simulink model "MultiLoop_mode1"  (R2021b)
settings: Solver=ode45  StartTime=0.0  StopTime=72  FixedStep=Ts_base  MinStep=1e-6  RelTol=1e-6
PreLoadFcn:
  | Mode_1_Init
InitFcn:
  | hApp = TEP_app;
  | %hApp = fault_selection_App;
StartFcn:
  | disp('simulator')
  | blk = 'MultiLoop_mode1/TE Plant/Pressure';
  | event = 'PostOutputs';
  | listener = @(app, event) updateGUI(hApp);
  | h = add_exec_event_listener(blk, event, listener);
StopFcn:
  | %TEplot
undefined symbols (not defined in the file or in its folder): Eadj_0, r1_0, r4_0, r5_0, r6_0, r7_0, SP17_0, Ts_base, Ts_save, xmv10_0, xmv11_0
libraries: TElib x8
settings Model: Creator=ricker  LastModifiedBy=kaung
settings SolverCC: AlgebraicLoopSolver=TrustRegion
settings DataIOCC: LoadInitialState=on  SaveFinalState=on  SaveFormat=Structure  SignalLoggingSaveFormat=ModelDataLogs  SaveOutput=off  SignalLogging=off  SaveTime=off  ReturnWorkspaceOutputs=off  SignalLoggingName=sigsOut
settings OptimizationCC: InitFltsAndDblsToZero=on  LifeSpan=inf
settings DebuggingCC: SaveWithParameterizedLinksMsg=none  UnderspecifiedInitializationDetection=Classic  MergeDetectMultiDrivingBlocksExec=none  SignalResolutionControl=TryResolveAllWithWarning  MultiTaskDSMMsg=warning  MultiTaskCondExecSysMsg=none  FcnCallInpInsideContextMsg=warning  SFUnexpectedBacktrackingDiag=warning  SFNoUnconditionalDefaultTransitionDiag=warning  SFExecutionAtInitializationDiag=none  SFMachineParentedDataDiag=warning  ArithmeticOperatorsInVariantConditions=warning
settings HardwareCC: ProdBitPerPointer=32  ProdBitPerSizeT=32  ProdBitPerPtrDiffT=32  ProdLargestAtomicFloat=None  ProdIntDivRoundTo=Undefined  ProdEndianess=Unspecified  ProdWordSize=32  ProdHWDeviceType=32-bit Generic  TargetUnknown=on
settings ModelReferenceCC: PropagateSignalLabelsOutOfModel=off
settings SFSimCC: SimUseLocalCustomCode=off  CustomCodeUndefinedFunction=UseInterfaceOnly
settings RTWCC: RTWUseLocalCustomCode=off
settings CodeAppCC: StateflowObjectComments=on
settings GRTTargetCC: TargetFcnLib=ansi_tfl_tmw.mat  TargetLangStandard=C89/C90 (ANSI)  CombineOutputUpdateFcns=off  GRTInterface=on
settings ConfigComp: CovMetricSettings=dw  CovSaveCumulativeToWorkspaceVar=on  CovSaveSingleToWorkspaceVar=on  CovExternalEMLEnable=off  CovSFcnEnable=off

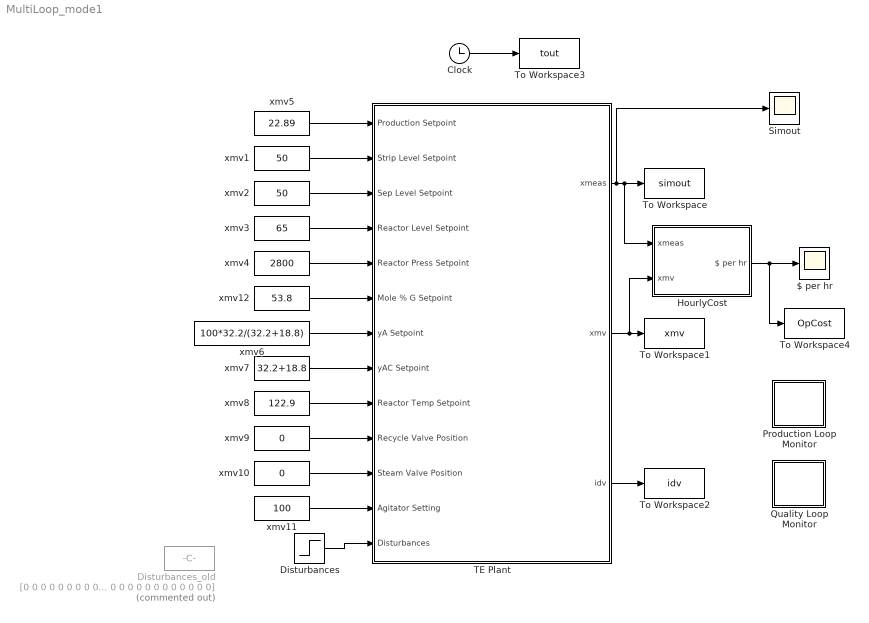
== system MultiLoop_mode1 ==
  $ per hr : Scope
  Clock : Clock
  Disturbances : Step  Time=0  Before=[0 0 0 0 0 0 0 0 0 0 0 0 0 0 0 0 0 0 0 0 0 0 0 0 0 0 0 0]  After=[1 0 0 0 0 0 0 0 0 0 0 0 0 0 0 0 0 0 0 0 0 0 0 0 0 0 0 0]  SampleTime=0
  Disturbances_old : Constant  Commented=on  Value=[0 0 0 0 0 0 0 0 0 0 0 0 0 0 0 0 0 0 0 0 0 0 0 0 0 0 0 0]
  HourlyCost : Subsystem
  Production Loop Monitor : Subsystem
  Quality Loop Monitor : Subsystem
  Simout : Scope
  TE Plant : Subsystem
  To Workspace : ToWorkspace  VariableName=simout  SampleTime=Ts_save
  To Workspace1 : ToWorkspace  VariableName=xmv  SampleTime=Ts_save
  To Workspace2 : ToWorkspace  VariableName=idv  SampleTime=Ts_save
  To Workspace3 : ToWorkspace  VariableName=tout  SampleTime=Ts_save
  To Workspace4 : ToWorkspace  VariableName=OpCost  SampleTime=Ts_save
  xmv1 : Constant  Value=50
  xmv10 : Constant  Value=0
  xmv11 : Constant  Value=100
  xmv12 : Constant  Value=53.8
  xmv2 : Constant  Value=50
  xmv3 : Constant  Value=65
  xmv4 : Constant  Value=2800
  xmv5 : Constant  Value=22.89
  xmv6 : Constant  Value=100*32.2/(32.2+18.8)
  xmv7 : Constant  Value=32.2+18.8
  xmv8 : Constant  Value=122.9
  xmv9 : Constant  Value=0
  wires:
  TE Plant/1(xmeas) -> Simout/1, To Workspace/1, HourlyCost/1(xmeas)
  xmv1/1 -> TE Plant/2(Strip Level Setpoint)
  xmv2/1 -> TE Plant/3(Sep Level Setpoint)
  xmv3/1 -> TE Plant/4(Reactor Level Setpoint)
  xmv4/1 -> TE Plant/5(Reactor Press Setpoint)
  xmv8/1 -> TE Plant/9(Reactor Temp Setpoint)
  xmv6/1 -> TE Plant/7(yA Setpoint)
  xmv7/1 -> TE Plant/8(yAC Setpoint)
  TE Plant/2(xmv) -> To Workspace1/1, HourlyCost/2(xmv)
  TE Plant/3(idv) -> To Workspace2/1
  Clock/1 -> To Workspace3/1
  HourlyCost/1($ per hr) -> $ per hr/1, To Workspace4/1
  xmv9/1 -> TE Plant/10(Recycle Valve Position)
  xmv10/1 -> TE Plant/11(Steam Valve Position)
  xmv11/1 -> TE Plant/12(Agitator Setting)
  xmv12/1 -> TE Plant/6(Mole % G Setpoint)
  Disturbances/1 -> TE Plant/13(Disturbances)
  xmv5/1 -> TE Plant/1(Production Setpoint)

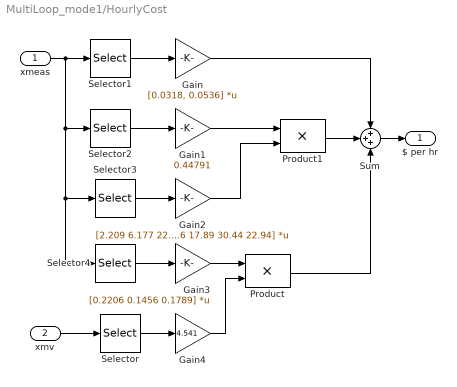
== system MultiLoop_mode1/HourlyCost ==
  xmeas : Inport  PortDimensions=41
  xmv : Inport  Port=2  PortDimensions=12
  Gain : Gain  Gain=[0.0318, 0.0536]  Multiplication=Matrix(K*u)  SaturateOnIntegerOverflow=on  OutDataTypeStr=Inherit: Same as input  ParamDataTypeStr=Inherit: Same as input
  Gain1 : Gain  Gain=0.44791  SaturateOnIntegerOverflow=on  OutDataTypeStr=Inherit: Same as input  ParamDataTypeStr=Inherit: Same as input
  Gain2 : Gain  Gain=[2.209 6.177 22.06 14.56 17.89 30.44 22.94]  Multiplication=Matrix(K*u)  SaturateOnIntegerOverflow=on  OutDataTypeStr=Inherit: Same as input  ParamDataTypeStr=Inherit: Same as input
  Gain3 : Gain  Gain=[0.2206 0.1456 0.1789]  Multiplication=Matrix(K*u)  SaturateOnIntegerOverflow=on  OutDataTypeStr=Inherit: Same as input  ParamDataTypeStr=Inherit: Same as input
  Gain4 : Gain  Gain=4.541  SaturateOnIntegerOverflow=on  OutDataTypeStr=Inherit: Same as input  ParamDataTypeStr=Inherit: Same as input
  Product : Product  SaturateOnIntegerOverflow=on  OutDataTypeStr=Inherit: Same as first input
  Product1 : Product  SaturateOnIntegerOverflow=on  OutDataTypeStr=Inherit: Same as first input
  Selector : Selector  InputPortWidth=12  IndexOptions=Index vector (dialog)  Indices=8  OutputSizes=1
  Selector1 : Selector  InputPortWidth=41  IndexOptions=Index vector (dialog)  Indices=[19 20]  OutputSizes=1
  Selector2 : Selector  InputPortWidth=41  IndexOptions=Index vector (dialog)  Indices=[10]  OutputSizes=1
  Selector3 : Selector  InputPortWidth=41  IndexOptions=Index vector (dialog)  Indices=[29, 31:36]  OutputSizes=1
  Selector4 : Selector  InputPortWidth=41  IndexOptions=Index vector (dialog)  Indices=[37:39]  OutputSizes=1
  Sum : Sum  Inputs=+++  SaturateOnIntegerOverflow=on
  $ per hr : Outport
  wires:
  xmv/1 -> Selector/1
  xmeas/1 -> Selector1/1, Selector2/1, Selector3/1, Selector4/1
  Selector1/1 -> Gain/1
  Selector2/1 -> Gain1/1
  Selector3/1 -> Gain2/1
  Selector4/1 -> Gain3/1
  Selector/1 -> Gain4/1
  Gain3/1 -> Product/1
  Gain4/1 -> Product/2
  Sum/1 -> $ per hr/1
  Product/1 -> Sum/3
  Gain/1 -> Sum/1
  Product1/1 -> Sum/2
  Gain1/1 -> Product1/1
  Gain2/1 -> Product1/2

== system MultiLoop_mode1/Production Loop Monitor ==
  Mux2 : Mux  Inputs=2
  Production : Scope
  wires:
  Mux2/1 -> Production/1
  [xmeas17] -> Mux2/2
  [Prodsp] -> Mux2/1

== system MultiLoop_mode1/Quality Loop Monitor ==
  Mux2 : Mux  Inputs=2
  Quality : Scope
  wires:
  [PctGsp] -> Mux2/1
  [xmeas40] -> Mux2/2
  Mux2/1 -> Quality/1

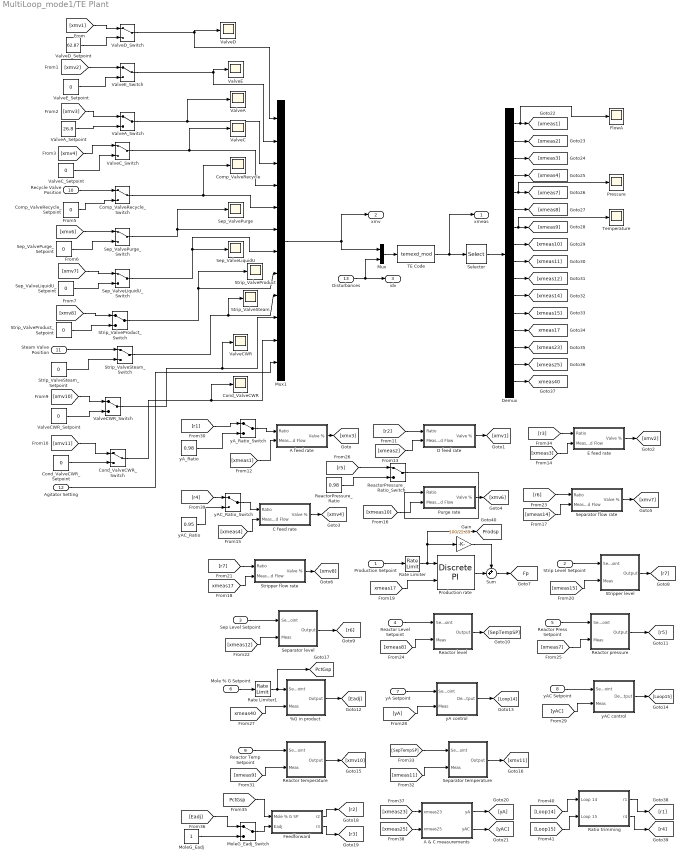
== system MultiLoop_mode1/TE Plant ==
  Production Setpoint : Inport
  Strip Level Setpoint : Inport  Port=2
  Sep Level Setpoint : Inport  Port=3
  Reactor Level Setpoint : Inport  Port=4
  Reactor Press Setpoint : Inport  Port=5
  Mole % G Setpoint : Inport  Port=6
  yA Setpoint : Inport  Port=7
  yAC Setpoint : Inport  Port=8
  Reactor Temp Setpoint : Inport  Port=9
  Recycle Valve Position : Inport  Port=10
  Steam Valve Position : Inport  Port=11
  Agitator Setting : Inport  Port=12
  Disturbances : Inport  Port=13
  %G in product : Subsystem  AncestorBlock=TElib/Discrete PI  mask{Kc=-0.4, Ti=100/60, Ts=Ts_base, x0=Eadj_0, Hi=inf, Lo=-inf}
  A & C measurements : Subsystem
  A feed rate : Subsystem
  C feed rate : Subsystem
  Comp_ValveRecycle : Scope
  Comp_ValveRecycle_Setpoint : Constant  Value=0
  Comp_ValveRecycle_Switch : ManualSwitch
  Cond_ValveCWR : Scope
  Cond_ValveCWR_Setpoint : Constant  Value=0
  Cond_ValveCWR_Switch : ManualSwitch
  D feed rate : Subsystem
  Demux : Demux  Outputs=16
      settings: DisplayOption=none
  E feed rate : Subsystem
  Feedforward : Subsystem
  FlowA : Scope
  Gain : Gain  Gain=100/22.89  SaturateOnIntegerOverflow=on  OutDataTypeStr=Inherit: Same as input  ParamDataTypeStr=Inherit: Same as input
  MoleG_Eadj : Constant
  MoleG_Eadj_Switch : ManualSwitch
  Mux : Mux  Inputs=2
  Mux1 : Mux  Inputs=12
  Pressure : Scope
  Production rate : TElib/Discrete PI  Kc=3.2  Ti=120/60  Ts=Ts_base  x0=0  Hi=30  Lo=-30
  Purge rate : Subsystem
  Rate Limiter : RateLimiter  RisingSlewLimit=0.3*22.95/24  FallingSlewLimit=-0.3*22.95/24
  Rate Limiter1 : RateLimiter  RisingSlewLimit=50/24  FallingSlewLimit=-50/24
  Ratio trimming : Subsystem
  Reactor level : Subsystem  AncestorBlock=TElib/Discrete PI  mask{Kc=0.8, Ti=60/60, Ts=Ts_base, x0=SP17_0, Hi=120, Lo=0}
  Reactor pressure : Subsystem  AncestorBlock=TElib/Discrete PI  mask{Kc=-1e-4, Ti=20/60, Ts=Ts_base, x0=r5_0, Hi=100, Lo=0}
  Reactor temperature : Subsystem  AncestorBlock=TElib/Discrete PI  mask{Kc=-8, Ti=7.5/60, Ts=Ts_base, x0=xmv10_0, Hi=100, Lo=0}
  ReactorPressure_Ratio : Constant  Value=0.98
  ReactorPressure_Ratio_Switch : ManualSwitch
  Selector : Selector  InputPortWidth=41  IndexOptions=Index vector (dialog)  Indices=[1:4, 7:12, 14, 15, 17, 23, 25, 40]  OutputSizes=1
  Sep_ValveLiquidU : Scope
  Sep_ValveLiquidU_Setpoint : Constant  Value=0
  Sep_ValveLiquidU_Switch : ManualSwitch
  Sep_ValvePurge : Scope
  Sep_ValvePurge_Setpoint : Constant  Value=0
  Sep_ValvePurge_Switch : ManualSwitch
  Separator flow rate : Subsystem
  Separator level : Subsystem  AncestorBlock=TElib/Discrete PI  mask{Kc=-1e-3, Ti=200/60, Ts=Ts_base, x0=r6_0, Hi=100, Lo=0}
  Separator temperature : Subsystem  AncestorBlock=TElib/Discrete PI  mask{Kc=-4, Ti=15/60, Ts=Ts_base, x0=xmv11_0, Hi=100, Lo=0}
  Strip_ValveProduct : Scope
  Strip_ValveProduct_Setpoint : Constant  Value=0
  Strip_ValveProduct_Switch : ManualSwitch
  Strip_ValveSteam : Scope
  Strip_ValveSteam_Setpoint : Constant  Value=0
  Strip_ValveSteam_Switch : ManualSwitch
  Stripper flow rate : Subsystem
  Stripper level : Subsystem  AncestorBlock=TElib/Discrete PI  mask{Kc=-2e-4, Ti=200/60, Ts=Ts_base, x0=r7_0, Hi=100, Lo=0}
  Sum : Sum  Inputs=++|  SaturateOnIntegerOverflow=on
  TE Code : S-Function  FunctionName=temexd_mod  SFunctionDeploymentMode=off  EnableBusSupport=off
  Temperature : Scope
  ValveA : Scope
  ValveA_Setpoint : Constant  Value=26.8
  ValveA_Switch : ManualSwitch
  ValveC : Scope
  ValveCWR : Scope
  ValveCWR_Setpoint : Constant  Value=0
  ValveCWR_Switch : ManualSwitch
  ValveC_Setpoint : Constant  Value=0
  ValveC_Switch : ManualSwitch
  ValveD : Scope
  ValveD_Setpoint : Constant  Value=62.87
  ValveD_Switch : ManualSwitch
  ValveE : Scope
  ValveE_Setpoint : Constant  Value=0
  ValveE_Switch : ManualSwitch
  yA control : Subsystem  AncestorBlock=TElib/Discrete PI/Vel PI  mask{Kc=2e-4, Ti=1, Ts=0.1}
  yAC control : Subsystem  AncestorBlock=TElib/Discrete PI/Vel PI  mask{Kc=3e-4, Ti=2, Ts=0.1}
  yAC_Ratio : Constant  Value=0.95
  yAC_Ratio_Switch : ManualSwitch
  yA_Ratio : Constant  Value=0.98
  yA_Ratio_Switch : ManualSwitch
  xmeas : Outport
  xmv : Outport  Port=2
  idv : Outport  Port=3
  tag scope: Fp=global, PctGsp=global, Prodsp=global, xmeas17=global, xmeas40=global
  wires:
  Mux/1 -> TE Code/1
  Disturbances/1 -> Mux/2, idv/1
  TE Code/1 -> xmeas/1, Selector/1
  [xmv1] -> ValveD_Switch/1
  Recycle Valve Position/1 -> Comp_ValveRecycle_Switch/1
  [xmv6] -> Sep_ValvePurge_Switch/1
  [xmv7] -> Sep_ValveLiquidU_Switch/1
  [xmv8] -> Strip_ValveProduct_Switch/1
  Steam Valve Position/1 -> Strip_ValveSteam_Switch/1
  [xmv10] -> ValveCWR_Switch/1
  [xmv11] -> Cond_ValveCWR_Switch/1
  Agitator Setting/1 -> Mux1/12
  A feed rate/1(Valve %) -> [xmv3]
  [xmeas1] -> A feed rate/2(Measured Flow)
  D feed rate/1(Valve %) -> [xmv1]
  [xmeas2] -> D feed rate/2(Measured Flow)
  E feed rate/1(Valve %) -> [xmv2]
  [xmeas3] -> E feed rate/2(Measured Flow)
  C feed rate/1(Valve %) -> [xmv4]
  [xmeas4] -> C feed rate/2(Measured Flow)
  Purge rate/1(Valve %) -> [xmv6]
  [xmeas10] -> Purge rate/2(Measured Flow)
  Separator flow rate/1(Valve %) -> [xmv7]
  [xmeas14] -> Separator flow rate/2(Measured Flow)
  Stripper flow rate/1(Valve %) -> [xmv8]
  [xmeas17] -> Stripper flow rate/2(Measured Flow)
  [xmeas17] -> Production rate/2
  [xmeas15] -> Stripper level/2(Meas)
  Strip Level Setpoint/1 -> Stripper level/1(Setpoint)
  Stripper level/1(Output) -> [r7]
  [r7] -> Stripper flow rate/1(Ratio)
  [xmeas12] -> Separator level/2(Meas)
  Sep Level Setpoint/1 -> Separator level/1(Setpoint)
  Separator level/1(Output) -> [r6]
  [r6] -> Separator flow rate/1(Ratio)
  [xmeas8] -> Reactor level/2(Meas)
  Reactor Level Setpoint/1 -> Reactor level/1(Setpoint)
  Reactor level/1(Output) -> [SepTempSP]
  [xmeas7] -> Reactor pressure/2(Meas)
  Reactor Press Setpoint/1 -> Reactor pressure/1(Setpoint)
  Reactor pressure/1(Output) -> [r5]
  [r5] -> ReactorPressure_Ratio_Switch/1
  [xmeas40] -> %G in product/2(Meas)
  %G in product/1(Output) -> [Eadj]
  [yA] -> yA control/2(Meas)
  yA Setpoint/1 -> yA control/1(Setpoint)
  yA control/1(Delta Output) -> [Loop14]
  [yAC] -> yAC control/2(Meas)
  yAC Setpoint/1 -> yAC control/1(Setpoint)
  yAC control/1(Delta Output) -> [Loop15]
  [r1] -> yA_Ratio_Switch/1
  [xmeas9] -> Reactor temperature/2(Meas)
  Reactor Temp Setpoint/1 -> Reactor temperature/1(Setpoint)
  Reactor temperature/1(Output) -> [xmv10]
  [xmeas11] -> Separator temperature/2(Meas)
  [SepTempSP] -> Separator temperature/1(Setpoint)
  Separator temperature/1(Output) -> [xmv11]
  [r3] -> E feed rate/1(Ratio)
  [PctGsp] -> Feedforward/1(Mole % G SP)
  [Eadj] -> MoleG_Eadj_Switch/1
  Feedforward/1(r2) -> [r2]
  Feedforward/2(r3) -> [r3]
  [xmeas23] -> A & C measurements/1(xmeas23)
  [xmeas25] -> A & C measurements/2(xmeas25)
  A & C measurements/1(yA) -> [yA]
  A & C measurements/2(yAC) -> [yAC]
  Mux1/1 -> Mux/1, xmv/1
  Selector/1 -> Demux/1
  Demux/1 -> FlowA/1, [xmeas1]
  Demux/2 -> [xmeas2]
  Demux/3 -> [xmeas3]
  Demux/4 -> [xmeas4]
  Demux/5 -> [xmeas7], Pressure/1
  Demux/6 -> [xmeas8]
  Demux/7 -> [xmeas9], Temperature/1
  Demux/8 -> [xmeas10]
  Demux/9 -> [xmeas11]
  Demux/10 -> [xmeas12]
  Demux/11 -> [xmeas14]
  Demux/12 -> [xmeas15]
  Demux/13 -> [xmeas17]
  Demux/14 -> [xmeas23]
  Demux/15 -> [xmeas25]
  Demux/16 -> [xmeas40]
  [r4] -> yAC_Ratio_Switch/1
  [Loop14] -> Ratio trimming/1(Loop 14)
  [Loop15] -> Ratio trimming/2(Loop 15)
  Ratio trimming/1(r1) -> [r1]
  Ratio trimming/2(r4) -> [r4]
  Production Setpoint/1 -> Rate Limiter/1
  Rate Limiter/1 -> Production rate/1, [Prodsp], Gain/1
  Mole % G Setpoint/1 -> Rate Limiter1/1
  Rate Limiter1/1 -> %G in product/1(Setpoint), [PctGsp]
  Production rate/1 -> Sum/2
  Sum/1 -> [Fp]
  Gain/1 -> Sum/1
  ValveD_Setpoint/1 -> ValveD_Switch/2
  ValveD_Switch/1 -> Mux1/1, ValveD/1
  Cond_ValveCWR_Setpoint/1 -> Cond_ValveCWR_Switch/2
  Cond_ValveCWR_Switch/1 -> Cond_ValveCWR/1, Mux1/11
  Sep_ValvePurge_Setpoint/1 -> Sep_ValvePurge_Switch/2
  Sep_ValvePurge_Switch/1 -> Mux1/6, Sep_ValvePurge/1
  Sep_ValveLiquidU_Setpoint/1 -> Sep_ValveLiquidU_Switch/2
  Sep_ValveLiquidU_Switch/1 -> Mux1/7, Sep_ValveLiquidU/1
  Comp_ValveRecycle_Switch/1 -> Comp_ValveRecycle/1, Mux1/5
  Comp_ValveRecycle_Setpoint/1 -> Comp_ValveRecycle_Switch/2
  [xmv3] -> ValveA_Switch/1
  ValveA_Switch/1 -> Mux1/3, ValveA/1
  ValveA_Setpoint/1 -> ValveA_Switch/2
  ValveE_Switch/1 -> Mux1/2, ValveE/1
  [xmv2] -> ValveE_Switch/1
  [xmv4] -> ValveC_Switch/1
  ValveC_Switch/1 -> ValveC/1, Mux1/4
  ValveC_Setpoint/1 -> ValveC_Switch/2
  Strip_ValveProduct_Setpoint/1 -> Strip_ValveProduct_Switch/2
  Strip_ValveProduct_Switch/1 -> Strip_ValveProduct/1, Mux1/8
  ValveCWR_Setpoint/1 -> ValveCWR_Switch/2
  ValveCWR_Switch/1 -> ValveCWR/1, Mux1/10
  Strip_ValveSteam_Switch/1 -> Strip_ValveSteam/1, Mux1/9
  Strip_ValveSteam_Setpoint/1 -> Strip_ValveSteam_Switch/2
  ValveE_Setpoint/1 -> ValveE_Switch/2
  [r2] -> D feed rate/1(Ratio)
  ReactorPressure_Ratio/1 -> ReactorPressure_Ratio_Switch/2
  ReactorPressure_Ratio_Switch/1 -> Purge rate/1(Ratio)
  MoleG_Eadj/1 -> MoleG_Eadj_Switch/2
  MoleG_Eadj_Switch/1 -> Feedforward/2(Eadj)
  yA_Ratio/1 -> yA_Ratio_Switch/2
  yA_Ratio_Switch/1 -> A feed rate/1(Ratio)
  yAC_Ratio/1 -> yAC_Ratio_Switch/2
  yAC_Ratio_Switch/1 -> C feed rate/1(Ratio)

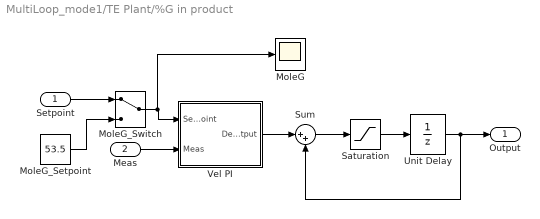
== system MultiLoop_mode1/TE Plant/%G in product ==
  Setpoint : Inport
  Meas : Inport  Port=2
  MoleG : Scope
  MoleG_Setpoint : Constant  Value=53.5
  MoleG_Switch : ManualSwitch
  Saturation : Saturate  UpperLimit=Hi  LowerLimit=Lo
  Sum : Sum  Inputs=|++  SaturateOnIntegerOverflow=on
  Unit Delay : UnitDelay  InitialCondition=x0  SampleTime=Ts
  Vel PI : Subsystem  mask{Kc=Kc, Ti=Ti, Ts=Ts}
  Output : Outport
  wires:
  Setpoint/1 -> MoleG_Switch/1
  Meas/1 -> Vel PI/2(Meas)
  Unit Delay/1 -> Output/1, Sum/2
  Saturation/1 -> Unit Delay/1
  Vel PI/1(Delta Output) -> Sum/1
  Sum/1 -> Saturation/1
  MoleG_Setpoint/1 -> MoleG_Switch/2
  MoleG_Switch/1 -> MoleG/1, Vel PI/1(Setpoint)

== system MultiLoop_mode1/TE Plant/A & C measurements ==
  xmeas23 : Inport
  xmeas25 : Inport  Port=2
  Gain1 : Gain  Gain=100  SaturateOnIntegerOverflow=on  OutDataTypeStr=Inherit: Same as input  ParamDataTypeStr=Inherit: Same as input
  Product1 : Product  Inputs=*/  SaturateOnIntegerOverflow=on  OutDataTypeStr=Inherit: Same as first input
  Sum1 : Sum  Inputs=++|  SaturateOnIntegerOverflow=on
  yA : Outport
  yAC : Outport  Port=2
  wires:
  Sum1/1 -> yAC/1, Product1/2
  xmeas23/1 -> Sum1/1, Gain1/1
  xmeas25/1 -> Sum1/2
  Gain1/1 -> Product1/1
  Product1/1 -> yA/1

== system MultiLoop_mode1/TE Plant/A feed rate ==
  Ratio : Inport
  Measured Flow : Inport  Port=2
  A_Feed : Scope
  A_Feed_Setpoint : Constant  Value=0.01
  A_Feed_Switch : ManualSwitch
  Discrete PI : TElib/Discrete PI  Kc=0.01  Ti=0.001/60  Ts=Ts_base  x0=xmv3_0  Hi=100  Lo=0
  Product : Product  SaturateOnIntegerOverflow=on  OutDataTypeStr=Inherit: Same as first input
  Valve % : Outport
  wires:
  Discrete PI/1 -> Valve %/1
  Ratio/1 -> Product/1
  [Fp] -> Product/2
  Measured Flow/1 -> Discrete PI/2
  Product/1 -> A_Feed_Switch/1
  A_Feed_Setpoint/1 -> A_Feed_Switch/2
  A_Feed_Switch/1 -> Discrete PI/1, A_Feed/1

== system MultiLoop_mode1/TE Plant/C feed rate ==
  Ratio : Inport
  Measured Flow : Inport  Port=2
  C_Feed : Scope
  C_Feed_Setpoint : Constant  Value=2
  C_Feed_Switch : ManualSwitch
  Discrete PI : TElib/Discrete PI  Kc=0.003  Ti=0.001/60  Ts=Ts_base  x0=xmv4_0  Hi=100  Lo=0
  Product : Product  SaturateOnIntegerOverflow=on  OutDataTypeStr=Inherit: Same as first input
  Valve % : Outport
  wires:
  Product/1 -> C_Feed_Switch/1
  Measured Flow/1 -> Discrete PI/2
  [Fp] -> Product/2
  Ratio/1 -> Product/1
  Discrete PI/1 -> Valve %/1
  C_Feed_Setpoint/1 -> C_Feed_Switch/2
  C_Feed_Switch/1 -> C_Feed/1, Discrete PI/1

== system MultiLoop_mode1/TE Plant/D feed rate ==
  Ratio : Inport
  Measured Flow : Inport  Port=2
  D_Feed : Scope
  D_Feed_Setpoint : Constant  Value=3
  D_Feed_Switch : ManualSwitch
  Discrete PI : TElib/Discrete PI  Kc=1.6e-6  Ti=0.001/60  Ts=Ts_base  x0=xmv1_0  Hi=100  Lo=0
  Product : Product  SaturateOnIntegerOverflow=on  OutDataTypeStr=Inherit: Same as first input
  Valve % : Outport
  wires:
  Product/1 -> D_Feed_Switch/1
  Measured Flow/1 -> Discrete PI/2
  [Fp] -> Product/2
  Ratio/1 -> Product/1
  Discrete PI/1 -> Valve %/1
  D_Feed_Setpoint/1 -> D_Feed_Switch/2
  D_Feed_Switch/1 -> D_Feed/1, Discrete PI/1

== system MultiLoop_mode1/TE Plant/E feed rate ==
  Ratio : Inport
  Measured Flow : Inport  Port=2
  Discrete PI : TElib/Discrete PI  Kc=1.8e-6  Ti=0.001/60  Ts=Ts_base  x0=xmv2_0  Hi=100  Lo=0
  E_Feed : Scope
  E_Feed_Setpoint : Constant
  E_Feed_Switch : ManualSwitch
  Product : Product  SaturateOnIntegerOverflow=on  OutDataTypeStr=Inherit: Same as first input
  Valve % : Outport
  wires:
  Product/1 -> E_Feed_Switch/1
  Measured Flow/1 -> Discrete PI/2
  [Fp] -> Product/2
  Ratio/1 -> Product/1
  Discrete PI/1 -> Valve %/1
  E_Feed_Switch/1 -> E_Feed/1, Discrete PI/1
  E_Feed_Setpoint/1 -> E_Feed_Switch/2

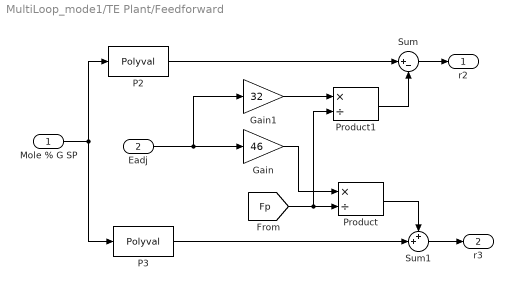
== system MultiLoop_mode1/TE Plant/Feedforward ==
  Mole % G SP : Inport
  Eadj : Inport  Port=2
  Gain : Gain  Gain=46  SaturateOnIntegerOverflow=on  OutDataTypeStr=Inherit: Same as input  ParamDataTypeStr=Inherit: Same as input
  Gain1 : Gain  Gain=32  SaturateOnIntegerOverflow=on  OutDataTypeStr=Inherit: Same as input  ParamDataTypeStr=Inherit: Same as input
  P2 : Polyval  Coefs="[1.5192e-003  5.9446e-001  2.7690e-001]"
  P3 : Polyval  Coefs="[-1.1377e-003 -8.0893e-001  9.1060e+001]"
  Product : Product  Inputs=*/  SaturateOnIntegerOverflow=on  OutDataTypeStr=Inherit: Same as first input
  Product1 : Product  Inputs=*/  SaturateOnIntegerOverflow=on  OutDataTypeStr=Inherit: Same as first input
  Sum : Sum  Inputs=|+-  SaturateOnIntegerOverflow=on
  Sum1 : Sum  Inputs=++|  SaturateOnIntegerOverflow=on
  r2 : Outport
  r3 : Outport  Port=2
  wires:
  Mole % G SP/1 -> P2/1, P3/1
  Sum/1 -> r2/1
  P2/1 -> Sum/1
  Sum1/1 -> r3/1
  P3/1 -> Sum1/2
  Product/1 -> Sum1/1
  [Fp] -> Product/2, Product1/2
  Gain/1 -> Product/1
  Eadj/1 -> Gain/1, Gain1/1
  Product1/1 -> Sum/2
  Gain1/1 -> Product1/1

== system MultiLoop_mode1/TE Plant/Purge rate ==
  Ratio : Inport
  Measured Flow : Inport  Port=2
  Discrete PI : TElib/Discrete PI  Kc=0.01  Ti=0.001/60  Ts=Ts_base  x0=xmv6_0  Hi=100  Lo=0
  Product : Product  SaturateOnIntegerOverflow=on  OutDataTypeStr=Inherit: Same as first input
  PurgeFlow : Scope
  PurgeFlow_Setpoint : Constant  Value=0.1
  PurgeFlow_Switch : ManualSwitch
  Valve % : Outport
  wires:
  Discrete PI/1 -> Valve %/1
  Ratio/1 -> Product/1
  [Fp] -> Product/2
  Measured Flow/1 -> Discrete PI/2
  Product/1 -> PurgeFlow_Switch/1
  PurgeFlow_Setpoint/1 -> PurgeFlow_Switch/2
  PurgeFlow_Switch/1 -> PurgeFlow/1, Discrete PI/1

== system MultiLoop_mode1/TE Plant/Ratio trimming ==
  Loop 14 : Inport
  Loop 15 : Inport  Port=2
  Sum1 : Sum  Inputs=-++  SaturateOnIntegerOverflow=on
  Sum2 : Sum  Inputs=++|  SaturateOnIntegerOverflow=on
  Unit Delay : UnitDelay  InitialCondition=r1_0  SampleTime=0.1  HasFrameUpgradeWarning=on
  Unit Delay1 : UnitDelay  InitialCondition=r4_0  SampleTime=0.1  HasFrameUpgradeWarning=on
  r1 : Outport
  r4 : Outport  Port=2
  wires:
  Loop 15/1 -> Sum1/2
  Unit Delay/1 -> Sum2/1
  Unit Delay1/1 -> Sum1/3
  Sum2/1 -> Unit Delay/1, r1/1
  Loop 14/1 -> Sum2/2, Sum1/1
  Sum1/1 -> Unit Delay1/1, r4/1

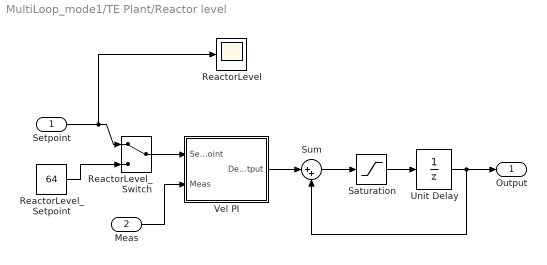
== system MultiLoop_mode1/TE Plant/Reactor level ==
  Setpoint : Inport
  Meas : Inport  Port=2
  ReactorLevel : Scope
  ReactorLevel_Setpoint : Constant  Value=64
  ReactorLevel_Switch : ManualSwitch
  Saturation : Saturate  UpperLimit=Hi  LowerLimit=Lo
  Sum : Sum  Inputs=|++  SaturateOnIntegerOverflow=on
  Unit Delay : UnitDelay  InitialCondition=x0  SampleTime=Ts
  Vel PI : Subsystem  mask{Kc=Kc, Ti=Ti, Ts=Ts}
  Output : Outport
  wires:
  Setpoint/1 -> ReactorLevel/1, ReactorLevel_Switch/1
  Meas/1 -> Vel PI/2(Meas)
  Unit Delay/1 -> Output/1, Sum/2
  Saturation/1 -> Unit Delay/1
  Vel PI/1(Delta Output) -> Sum/1
  Sum/1 -> Saturation/1
  ReactorLevel_Setpoint/1 -> ReactorLevel_Switch/2
  ReactorLevel_Switch/1 -> Vel PI/1(Setpoint)

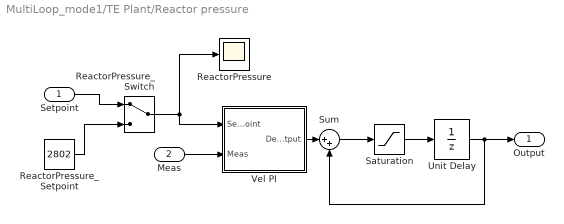
== system MultiLoop_mode1/TE Plant/Reactor pressure ==
  Setpoint : Inport
  Meas : Inport  Port=2
  ReactorPressure : Scope
  ReactorPressure_Setpoint : Constant  Value=2802
  ReactorPressure_Switch : ManualSwitch
  Saturation : Saturate  UpperLimit=Hi  LowerLimit=Lo
  Sum : Sum  Inputs=|++  SaturateOnIntegerOverflow=on
  Unit Delay : UnitDelay  InitialCondition=x0  SampleTime=Ts
  Vel PI : Subsystem  mask{Kc=Kc, Ti=Ti, Ts=Ts}
  Output : Outport
  wires:
  Setpoint/1 -> ReactorPressure_Switch/1
  Meas/1 -> Vel PI/2(Meas)
  Unit Delay/1 -> Output/1, Sum/2
  Saturation/1 -> Unit Delay/1
  Vel PI/1(Delta Output) -> Sum/1
  Sum/1 -> Saturation/1
  ReactorPressure_Setpoint/1 -> ReactorPressure_Switch/2
  ReactorPressure_Switch/1 -> Vel PI/1(Setpoint), ReactorPressure/1

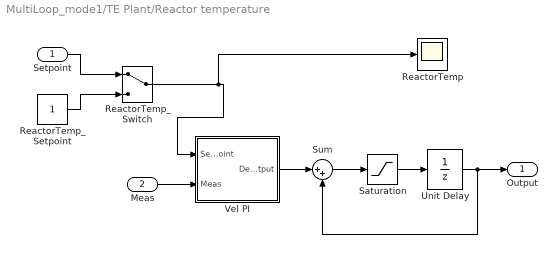
== system MultiLoop_mode1/TE Plant/Reactor temperature ==
  Setpoint : Inport
  Meas : Inport  Port=2
  ReactorTemp : Scope
  ReactorTemp_Setpoint : Constant
  ReactorTemp_Switch : ManualSwitch
  Saturation : Saturate  UpperLimit=Hi  LowerLimit=Lo
  Sum : Sum  Inputs=|++  SaturateOnIntegerOverflow=on
  Unit Delay : UnitDelay  InitialCondition=x0  SampleTime=Ts
  Vel PI : Subsystem  mask{Kc=Kc, Ti=Ti, Ts=Ts}
  Output : Outport
  wires:
  Setpoint/1 -> ReactorTemp_Switch/1
  Meas/1 -> Vel PI/2(Meas)
  Unit Delay/1 -> Output/1, Sum/2
  Saturation/1 -> Unit Delay/1
  Vel PI/1(Delta Output) -> Sum/1
  Sum/1 -> Saturation/1
  ReactorTemp_Setpoint/1 -> ReactorTemp_Switch/2
  ReactorTemp_Switch/1 -> ReactorTemp/1, Vel PI/1(Setpoint)

== system MultiLoop_mode1/TE Plant/Separator flow rate ==
  Ratio : Inport
  Measured Flow : Inport  Port=2
  Discrete PI : TElib/Discrete PI  Kc=4e-4  Ti=0.001/60  Ts=Ts_base  x0=xmv7_0  Hi=100  Lo=0
  Product : Product  SaturateOnIntegerOverflow=on  OutDataTypeStr=Inherit: Same as first input
  SepFlow : Scope
  SepFlow_Setpoint : Constant  Value=24.96
  SepFlow_Switch : ManualSwitch
  Valve % : Outport
  wires:
  Product/1 -> SepFlow_Switch/1
  Measured Flow/1 -> Discrete PI/2
  [Fp] -> Product/2
  Ratio/1 -> Product/1
  Discrete PI/1 -> Valve %/1
  SepFlow_Setpoint/1 -> SepFlow_Switch/2
  SepFlow_Switch/1 -> SepFlow/1, Discrete PI/1

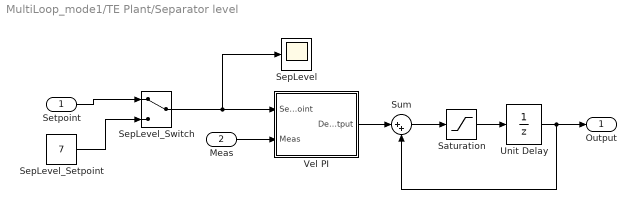
== system MultiLoop_mode1/TE Plant/Separator level ==
  Setpoint : Inport
  Meas : Inport  Port=2
  Saturation : Saturate  UpperLimit=Hi  LowerLimit=Lo
  SepLevel : Scope
  SepLevel_Setpoint : Constant  Value=7
  SepLevel_Switch : ManualSwitch
  Sum : Sum  Inputs=|++  SaturateOnIntegerOverflow=on
  Unit Delay : UnitDelay  InitialCondition=x0  SampleTime=Ts
  Vel PI : Subsystem  mask{Kc=Kc, Ti=Ti, Ts=Ts}
  Output : Outport
  wires:
  Setpoint/1 -> SepLevel_Switch/1
  Meas/1 -> Vel PI/2(Meas)
  Unit Delay/1 -> Output/1, Sum/2
  Saturation/1 -> Unit Delay/1
  Vel PI/1(Delta Output) -> Sum/1
  Sum/1 -> Saturation/1
  SepLevel_Setpoint/1 -> SepLevel_Switch/2
  SepLevel_Switch/1 -> SepLevel/1, Vel PI/1(Setpoint)

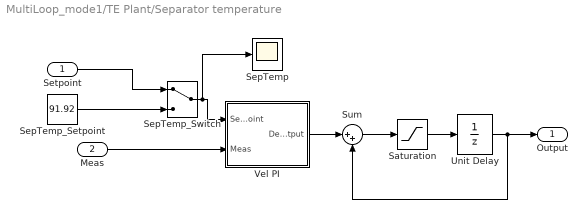
== system MultiLoop_mode1/TE Plant/Separator temperature ==
  Setpoint : Inport
  Meas : Inport  Port=2
  Saturation : Saturate  UpperLimit=Hi  LowerLimit=Lo
  SepTemp : Scope
  SepTemp_Setpoint : Constant  Value=91.92
  SepTemp_Switch : ManualSwitch
  Sum : Sum  Inputs=|++  SaturateOnIntegerOverflow=on
  Unit Delay : UnitDelay  InitialCondition=x0  SampleTime=Ts
  Vel PI : Subsystem  mask{Kc=Kc, Ti=Ti, Ts=Ts}
  Output : Outport
  wires:
  Setpoint/1 -> SepTemp_Switch/1
  Meas/1 -> Vel PI/2(Meas)
  Unit Delay/1 -> Output/1, Sum/2
  Saturation/1 -> Unit Delay/1
  Vel PI/1(Delta Output) -> Sum/1
  Sum/1 -> Saturation/1
  SepTemp_Setpoint/1 -> SepTemp_Switch/2
  SepTemp_Switch/1 -> SepTemp/1, Vel PI/1(Setpoint)

== system MultiLoop_mode1/TE Plant/Stripper flow rate ==
  Ratio : Inport
  Measured Flow : Inport  Port=2
  Discrete PI : TElib/Discrete PI  Kc=4e-4  Ti=0.001/60  Ts=Ts_base  x0=xmv8_0  Hi=100  Lo=0
  Product : Product  SaturateOnIntegerOverflow=on  OutDataTypeStr=Inherit: Same as first input
  ProductFlow : Scope
  ProductFlow_Setpoint : Constant  Value=1.4
  ProductFlow_Switch : ManualSwitch
  Valve % : Outport
  wires:
  Discrete PI/1 -> Valve %/1
  Ratio/1 -> Product/1
  [Fp] -> Product/2
  Measured Flow/1 -> Discrete PI/2
  Product/1 -> ProductFlow_Switch/1
  ProductFlow_Setpoint/1 -> ProductFlow_Switch/2
  ProductFlow_Switch/1 -> ProductFlow/1, Discrete PI/1

== system MultiLoop_mode1/TE Plant/Stripper level ==
  Setpoint : Inport
  Meas : Inport  Port=2
  Saturation : Saturate  UpperLimit=Hi  LowerLimit=Lo
  StripLevel : Scope
  StripLevel_Setpoint : Constant  Value=5
  StripLevel_Switch : ManualSwitch
  Sum : Sum  Inputs=|++  SaturateOnIntegerOverflow=on
  Unit Delay : UnitDelay  InitialCondition=x0  SampleTime=Ts
  Vel PI : Subsystem  mask{Kc=Kc, Ti=Ti, Ts=Ts}
  Output : Outport
  wires:
  Setpoint/1 -> StripLevel_Switch/1
  Meas/1 -> Vel PI/2(Meas)
  Unit Delay/1 -> Output/1, Sum/2
  Saturation/1 -> Unit Delay/1
  Vel PI/1(Delta Output) -> Sum/1
  Sum/1 -> Saturation/1
  StripLevel_Setpoint/1 -> StripLevel_Switch/2
  StripLevel_Switch/1 -> StripLevel/1, Vel PI/1(Setpoint)

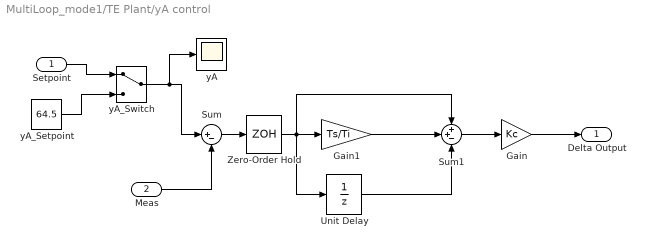
== system MultiLoop_mode1/TE Plant/yA control ==
  Setpoint : Inport
  Meas : Inport  Port=2
  Gain : Gain  Gain=Kc  SaturateOnIntegerOverflow=on  OutDataTypeStr=Inherit: Same as input  ParamDataTypeStr=Inherit: Same as input
  Gain1 : Gain  Gain=Ts/Ti  SaturateOnIntegerOverflow=on  OutDataTypeStr=Inherit: Same as input  ParamDataTypeStr=Inherit: Same as input
  Sum : Sum  Inputs=|+-  SaturateOnIntegerOverflow=on
  Sum1 : Sum  Inputs=++-  SaturateOnIntegerOverflow=on
  Unit Delay : UnitDelay  SampleTime=Ts
  Zero-Order Hold : ZeroOrderHold  SampleTime=Ts
  yA : Scope
  yA_Setpoint : Constant  Value=64.5
  yA_Switch : ManualSwitch
  Delta Output : Outport
  wires:
  Zero-Order Hold/1 -> Sum1/1, Unit Delay/1, Gain1/1
  Sum/1 -> Zero-Order Hold/1
  Unit Delay/1 -> Sum1/3
  Gain1/1 -> Sum1/2
  Sum1/1 -> Gain/1
  Gain/1 -> Delta Output/1
  Meas/1 -> Sum/2
  Setpoint/1 -> yA_Switch/1
  yA_Switch/1 -> yA/1, Sum/1
  yA_Setpoint/1 -> yA_Switch/2

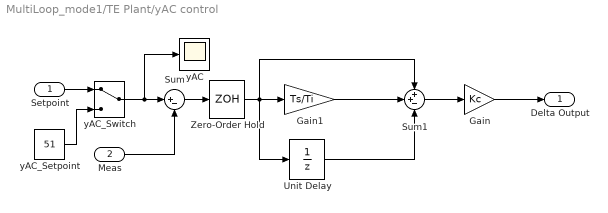
== system MultiLoop_mode1/TE Plant/yAC control ==
  Setpoint : Inport
  Meas : Inport  Port=2
  Gain : Gain  Gain=Kc  SaturateOnIntegerOverflow=on  OutDataTypeStr=Inherit: Same as input  ParamDataTypeStr=Inherit: Same as input
  Gain1 : Gain  Gain=Ts/Ti  SaturateOnIntegerOverflow=on  OutDataTypeStr=Inherit: Same as input  ParamDataTypeStr=Inherit: Same as input
  Sum : Sum  Inputs=|+-  SaturateOnIntegerOverflow=on
  Sum1 : Sum  Inputs=++-  SaturateOnIntegerOverflow=on
  Unit Delay : UnitDelay  SampleTime=Ts
  Zero-Order Hold : ZeroOrderHold  SampleTime=Ts
  yAC : Scope
  yAC_Setpoint : Constant  Value=51
  yAC_Switch : ManualSwitch
  Delta Output : Outport
  wires:
  Zero-Order Hold/1 -> Sum1/1, Unit Delay/1, Gain1/1
  Sum/1 -> Zero-Order Hold/1
  Unit Delay/1 -> Sum1/3
  Gain1/1 -> Sum1/2
  Sum1/1 -> Gain/1
  Gain/1 -> Delta Output/1
  Meas/1 -> Sum/2
  Setpoint/1 -> yAC_Switch/1
  yAC_Setpoint/1 -> yAC_Switch/2
  yAC_Switch/1 -> yAC/1, Sum/1

== system MultiLoop_mode1/TE Plant/%G in product/Vel PI ==
  Setpoint : Inport
  Meas : Inport  Port=2
  Gain : Gain  Gain=Kc  SaturateOnIntegerOverflow=on  OutDataTypeStr=Inherit: Same as input  ParamDataTypeStr=Inherit: Same as input
  Gain1 : Gain  Gain=Ts/Ti  SaturateOnIntegerOverflow=on  OutDataTypeStr=Inherit: Same as input  ParamDataTypeStr=Inherit: Same as input
  Sum : Sum  Inputs=|+-  SaturateOnIntegerOverflow=on
  Sum1 : Sum  Inputs=++-  SaturateOnIntegerOverflow=on
  Unit Delay : UnitDelay  SampleTime=Ts
  Zero-Order Hold : ZeroOrderHold  SampleTime=Ts
  Delta Output : Outport
  wires:
  Zero-Order Hold/1 -> Sum1/1, Unit Delay/1, Gain1/1
  Sum/1 -> Zero-Order Hold/1
  Unit Delay/1 -> Sum1/3
  Gain1/1 -> Sum1/2
  Sum1/1 -> Gain/1
  Gain/1 -> Delta Output/1
  Meas/1 -> Sum/2
  Setpoint/1 -> Sum/1

== system MultiLoop_mode1/TE Plant/Reactor level/Vel PI ==
  Setpoint : Inport
  Meas : Inport  Port=2
  Gain : Gain  Gain=Kc  SaturateOnIntegerOverflow=on  OutDataTypeStr=Inherit: Same as input  ParamDataTypeStr=Inherit: Same as input
  Gain1 : Gain  Gain=Ts/Ti  SaturateOnIntegerOverflow=on  OutDataTypeStr=Inherit: Same as input  ParamDataTypeStr=Inherit: Same as input
  Sum : Sum  Inputs=|+-  SaturateOnIntegerOverflow=on
  Sum1 : Sum  Inputs=++-  SaturateOnIntegerOverflow=on
  Unit Delay : UnitDelay  SampleTime=Ts
  Zero-Order Hold : ZeroOrderHold  SampleTime=Ts
  Delta Output : Outport
  wires:
  Zero-Order Hold/1 -> Sum1/1, Unit Delay/1, Gain1/1
  Sum/1 -> Zero-Order Hold/1
  Unit Delay/1 -> Sum1/3
  Gain1/1 -> Sum1/2
  Sum1/1 -> Gain/1
  Gain/1 -> Delta Output/1
  Meas/1 -> Sum/2
  Setpoint/1 -> Sum/1

== system MultiLoop_mode1/TE Plant/Reactor pressure/Vel PI ==
  Setpoint : Inport
  Meas : Inport  Port=2
  Gain : Gain  Gain=Kc  SaturateOnIntegerOverflow=on  OutDataTypeStr=Inherit: Same as input  ParamDataTypeStr=Inherit: Same as input
  Gain1 : Gain  Gain=Ts/Ti  SaturateOnIntegerOverflow=on  OutDataTypeStr=Inherit: Same as input  ParamDataTypeStr=Inherit: Same as input
  Sum : Sum  Inputs=|+-  SaturateOnIntegerOverflow=on
  Sum1 : Sum  Inputs=++-  SaturateOnIntegerOverflow=on
  Unit Delay : UnitDelay  SampleTime=Ts
  Zero-Order Hold : ZeroOrderHold  SampleTime=Ts
  Delta Output : Outport
  wires:
  Zero-Order Hold/1 -> Sum1/1, Unit Delay/1, Gain1/1
  Sum/1 -> Zero-Order Hold/1
  Unit Delay/1 -> Sum1/3
  Gain1/1 -> Sum1/2
  Sum1/1 -> Gain/1
  Gain/1 -> Delta Output/1
  Meas/1 -> Sum/2
  Setpoint/1 -> Sum/1

== system MultiLoop_mode1/TE Plant/Reactor temperature/Vel PI ==
  Setpoint : Inport
  Meas : Inport  Port=2
  Gain : Gain  Gain=Kc  SaturateOnIntegerOverflow=on  OutDataTypeStr=Inherit: Same as input  ParamDataTypeStr=Inherit: Same as input
  Gain1 : Gain  Gain=Ts/Ti  SaturateOnIntegerOverflow=on  OutDataTypeStr=Inherit: Same as input  ParamDataTypeStr=Inherit: Same as input
  Sum : Sum  Inputs=|+-  SaturateOnIntegerOverflow=on
  Sum1 : Sum  Inputs=++-  SaturateOnIntegerOverflow=on
  Unit Delay : UnitDelay  SampleTime=Ts
  Zero-Order Hold : ZeroOrderHold  SampleTime=Ts
  Delta Output : Outport
  wires:
  Zero-Order Hold/1 -> Sum1/1, Unit Delay/1, Gain1/1
  Sum/1 -> Zero-Order Hold/1
  Unit Delay/1 -> Sum1/3
  Gain1/1 -> Sum1/2
  Sum1/1 -> Gain/1
  Gain/1 -> Delta Output/1
  Meas/1 -> Sum/2
  Setpoint/1 -> Sum/1

== system MultiLoop_mode1/TE Plant/Separator level/Vel PI ==
  Setpoint : Inport
  Meas : Inport  Port=2
  Gain : Gain  Gain=Kc  SaturateOnIntegerOverflow=on  OutDataTypeStr=Inherit: Same as input  ParamDataTypeStr=Inherit: Same as input
  Gain1 : Gain  Gain=Ts/Ti  SaturateOnIntegerOverflow=on  OutDataTypeStr=Inherit: Same as input  ParamDataTypeStr=Inherit: Same as input
  Sum : Sum  Inputs=|+-  SaturateOnIntegerOverflow=on
  Sum1 : Sum  Inputs=++-  SaturateOnIntegerOverflow=on
  Unit Delay : UnitDelay  SampleTime=Ts
  Zero-Order Hold : ZeroOrderHold  SampleTime=Ts
  Delta Output : Outport
  wires:
  Zero-Order Hold/1 -> Sum1/1, Unit Delay/1, Gain1/1
  Sum/1 -> Zero-Order Hold/1
  Unit Delay/1 -> Sum1/3
  Gain1/1 -> Sum1/2
  Sum1/1 -> Gain/1
  Gain/1 -> Delta Output/1
  Meas/1 -> Sum/2
  Setpoint/1 -> Sum/1

== system MultiLoop_mode1/TE Plant/Separator temperature/Vel PI ==
  Setpoint : Inport
  Meas : Inport  Port=2
  Gain : Gain  Gain=Kc  SaturateOnIntegerOverflow=on  OutDataTypeStr=Inherit: Same as input  ParamDataTypeStr=Inherit: Same as input
  Gain1 : Gain  Gain=Ts/Ti  SaturateOnIntegerOverflow=on  OutDataTypeStr=Inherit: Same as input  ParamDataTypeStr=Inherit: Same as input
  Sum : Sum  Inputs=|+-  SaturateOnIntegerOverflow=on
  Sum1 : Sum  Inputs=++-  SaturateOnIntegerOverflow=on
  Unit Delay : UnitDelay  SampleTime=Ts
  Zero-Order Hold : ZeroOrderHold  SampleTime=Ts
  Delta Output : Outport
  wires:
  Zero-Order Hold/1 -> Sum1/1, Unit Delay/1, Gain1/1
  Sum/1 -> Zero-Order Hold/1
  Unit Delay/1 -> Sum1/3
  Gain1/1 -> Sum1/2
  Sum1/1 -> Gain/1
  Gain/1 -> Delta Output/1
  Meas/1 -> Sum/2
  Setpoint/1 -> Sum/1

== system MultiLoop_mode1/TE Plant/Stripper level/Vel PI ==
  Setpoint : Inport
  Meas : Inport  Port=2
  Gain : Gain  Gain=Kc  SaturateOnIntegerOverflow=on  OutDataTypeStr=Inherit: Same as input  ParamDataTypeStr=Inherit: Same as input
  Gain1 : Gain  Gain=Ts/Ti  SaturateOnIntegerOverflow=on  OutDataTypeStr=Inherit: Same as input  ParamDataTypeStr=Inherit: Same as input
  Sum : Sum  Inputs=|+-  SaturateOnIntegerOverflow=on
  Sum1 : Sum  Inputs=++-  SaturateOnIntegerOverflow=on
  Unit Delay : UnitDelay  SampleTime=Ts
  Zero-Order Hold : ZeroOrderHold  SampleTime=Ts
  Delta Output : Outport
  wires:
  Zero-Order Hold/1 -> Sum1/1, Unit Delay/1, Gain1/1
  Sum/1 -> Zero-Order Hold/1
  Unit Delay/1 -> Sum1/3
  Gain1/1 -> Sum1/2
  Sum1/1 -> Gain/1
  Gain/1 -> Delta Output/1
  Meas/1 -> Sum/2
  Setpoint/1 -> Sum/1
